simulink model "Problem3"  (R2014a)
settings: Solver=ode5  StartTime=0.0  StopTime=10.0  FixedStep=0.01  RelTol=1e-3
values from neighbouring files (symbols this model uses):
  ALa = [-0.2316 0.0633 -0.9956 0.0510; -29.4924 -3.0169 0.0201 0; 6.2346 -0.0274 -0.4169 0; 0 1 0.0631 0]    [Project_1.m]
  ALo = [-0.0111 -0.0788 -0.0033 -0.5615; -0.0092 -0.7531 0.9951 0; 0.0062 -1.5765 -0.7453 0; 0 0 1 0]    [Project_1.m]
  BLa = [0.0052 0.0310; -36.4909 8.1090; -0.4916 -2.8274; 0 0]    [Project_1.m]
  BLo = [0.0721; -0.1178; -9.0991; 0]    [Project_1.m]
  CLa = eye(4)    [Project_1.m]
  CLo = eye(4)    [Project_1.m]
  DLa = zeros(4,2)    [Project_1.m]
  DLo = zeros(4,1)    [Project_1.m]
settings Model: Creator=cmc4177  LastModifiedBy=cmc4177
settings DataIOCC: SaveOutput=off  SaveTime=off

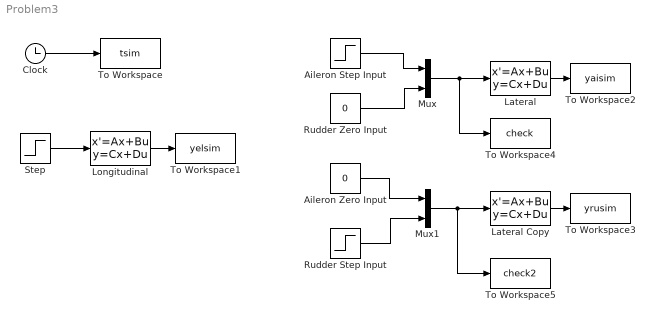
== system Problem3 ==
  Aileron Step Input : Step  After=-0.5  SampleTime=0
  Aileron Zero Input : Constant  Value=0
  Clock : Clock
  Lateral : StateSpace  A=ALa  B=BLa  C=CLa  D=DLa  X0=0
  Lateral Copy : StateSpace  A=ALa  B=BLa  C=CLa  D=DLa  X0=0
  Longitudinal : StateSpace  A=ALo  B=BLo  C=CLo  D=DLo  X0=0
  Mux : Mux  Inputs=2
  Mux1 : Mux  Inputs=2
  Rudder Step Input : Step  After=-0.5  SampleTime=0
  Rudder Zero Input : Constant  Value=0
  Step : Step  After=-0.5  SampleTime=0
  To Workspace : ToWorkspace  VariableName=tsim  SampleTime=-1
  To Workspace1 : ToWorkspace  VariableName=yelsim  SampleTime=-1
  To Workspace2 : ToWorkspace  VariableName=yaisim  SampleTime=-1
  To Workspace3 : ToWorkspace  VariableName=yrusim  SampleTime=-1
  To Workspace4 : ToWorkspace  VariableName=check  SampleTime=-1
  To Workspace5 : ToWorkspace  VariableName=check2  SampleTime=-1
  wires:
  Clock/1 -> To Workspace/1
  Aileron Zero Input/1 -> Mux1/1
  Rudder Step Input/1 -> Mux1/2
  Mux1/1 -> To Workspace5/1, Lateral Copy/1
  Rudder Zero Input/1 -> Mux/2
  Mux/1 -> To Workspace4/1, Lateral/1
  Aileron Step Input/1 -> Mux/1
  Step/1 -> Longitudinal/1
  Longitudinal/1 -> To Workspace1/1
  Lateral/1 -> To Workspace2/1
  Lateral Copy/1 -> To Workspace3/1
